simulink model "Controlador_NaoLinear_LQG"  (R2020a)
settings: Solver=ode8  StartTime=0.0  StopTime=50  FixedStep=0.01  RelTol=1e-3
values from neighbouring files (symbols this model uses):
  Ad = sysd.a    [Controlador.m]
  Bd = sysd.b    [Controlador.m]
  C = [1 0]    [Controlador.m]
  D = [0]    [Controlador.m]
  sysKFd = ss(Ad-Lf*C,[Bd Lf],eye(2),zeros(2,2))    [Controlador.m]
undefined symbols (not defined in the file or in its folder): kalmf, Krd
libraries: simulink x3
settings Model: Creator=Matheus  LastModifiedBy=mathe
settings DataIOCC: ReturnWorkspaceOutputs=off
settings DebuggingCC: ArithmeticOperatorsInVariantConditions=warning
settings SFSimCC: SimUseLocalCustomCode=off  CustomCodeUndefinedFunction=UseInterfaceOnly
settings RTWCC: RTWUseLocalCustomCode=off
settings CodeAppCC: StateflowObjectComments=on

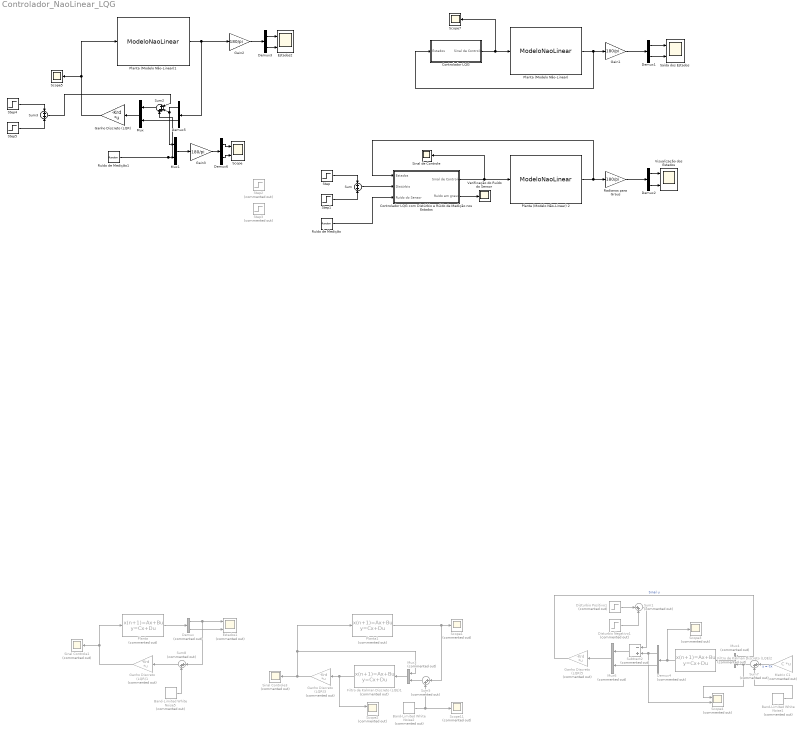
== system Controlador_NaoLinear_LQG ==
  Band-Limited White Noise1 : simulink/Sources/Band-Limited White Noise  Commented=on  Cov=0  Ts=0.05  seed=[23341]
  Band-Limited White Noise2 : simulink/Sources/Band-Limited White Noise  Commented=on  Cov=.0001  Ts=0.05  seed=[23341]
  Band-Limited White Noise5 : simulink/Sources/Band-Limited White Noise  Commented=on  Cov=.001  Ts=0.05  seed=[23341]
  Controlador LQG : Subsystem
  Controlador LQG com Distúrbio e Rúido de Medição nos Estados : Subsystem
  Demux : Demux  Commented=on  Outputs=2
  Demux{1..3,5..6} (5 alike) : Demux  Outputs=2
  Demux4 : Demux  Commented=on  Outputs=2
  Disturbio Negativo1 : Step  Commented=on  Time=10.5  After=-3.14/20
  Disturbio Positivo1 : Step  Commented=on  Time=10  After=3.14/20
  Estados1 : Scope  Commented=on  NumInputPorts=2
  Estados2 : Scope  NumInputPorts=2
  Filtro de Kalman Discreto (LQE)1 : DiscreteStateSpace  Commented=on  A=sysKFd.a  B=sysKFd.b  C=sysKFd.c  D=sysKFd.d  InitialCondition=[0 0]  SampleTime=0.05
  Filtro de Kalman Discreto (LQE)2 : DiscreteStateSpace  Commented=on  A=sysKFd.a  B=sysKFd.b  C=sysKFd.c  D=sysKFd.d  InitialCondition=[0 0]  SampleTime=-1
  Gain1 : Gain  Gain=180/pi
  Gain2 : Gain  Gain=180/pi
  Gain3 : Gain  Gain=180/pi
  Ganho Discreto (LQR) : Gain  Gain=-Krd  Multiplication=Matrix(K*u) (u vector)
  Ganho Discreto (LQR)1 : Gain  Commented=on  Gain=-Krd  Multiplication=Matrix(K*u) (u vector)
  Ganho Discreto (LQR)3 : Gain  Commented=on  Gain=-Krd  Multiplication=Matrix(K*u) (u vector)
  Ganho Discreto (LQR)5 : Gain  Commented=on  Gain=-Krd  Multiplication=Matrix(K*u) (u vector)
  Matriz C1 : Gain  Commented=on  Gain=C  Multiplication=Matrix(K*u) (u vector)
  Mux : Mux  Inputs=2
  Mux1 : Mux  Inputs=2
  Mux3 : Mux  Commented=on  Inputs=2
  Mux4 : Mux  Commented=on  Inputs=2
  Mux6 : Mux  Commented=on  Inputs=2
  Planta : DiscreteStateSpace  Commented=on  A=Ad  B=Bd  C=[eye(2); C]  D=[D; 0; 0]  InitialCondition=[pi/3 0]  SampleTime=0.05
  Planta (Modelo Não-Linear) : S-Function  InitFcn=try, set_param(gcb,'FunctionName','ModeloNaoLinear'), end  FunctionName=ModeloNaoLinear  SFunctionModules=ModeloNaoLinear_wrapper  SFunctionDeploymentMode=off  EnableBusSupport=off  mask(S-Function Builder){}
      mask help: Simulink:masks:SFunctionBuilder_MD
      mask init:
      | val = [[.9  0.75 0.75 1 1 .9 .9 1]',[1 1 0.75 0.75 .9 .9 1 .9]'];try , sys = get_param(gcb,'SfunBuilderFcnName');if isempty(sys), sys = get_param(gcb,'FunctionName'); end,catch, sys = get_param(gcb,'FunctionName'); end
      settings: CopyFcn=set_param(gcbh,'LinkStatus','none')  PreSaveFcn=try, set_param(gcb,'FunctionName','ModeloNaoLinear'), end  OpenFcn=sfunctionwizard(gcbh)
      mask Display: plot(val(:,1),val(:,2)),disp(sys), port_label('input',1,'u0'), port_label('output',1,'y0')
  Planta (Modelo Não-Linear) 2 : S-Function  InitFcn=try, set_param(gcb,'FunctionName','ModeloNaoLinear'), end  FunctionName=ModeloNaoLinear  SFunctionModules=ModeloNaoLinear_wrapper  SFunctionDeploymentMode=off  EnableBusSupport=off  mask(S-Function Builder){}
      mask help: Simulink:masks:SFunctionBuilder_MD
      mask init: same as Controlador_NaoLinear_LQG/Planta (Modelo Não-Linear)
      settings: CopyFcn=set_param(gcbh,'LinkStatus','none')  PreSaveFcn=try, set_param(gcb,'FunctionName','ModeloNaoLinear'), end  OpenFcn=sfunctionwizard(gcbh)
      mask Display: plot(val(:,1),val(:,2)),disp(sys), port_label('input',1,'u0'), port_label('output',1,'y0')
  Planta (Modelo Não-Linear)1 : S-Function  InitFcn=try, set_param(gcb,'FunctionName','ModeloNaoLinear'), end  FunctionName=ModeloNaoLinear  SFunctionModules=ModeloNaoLinear_wrapper  SFunctionDeploymentMode=off  EnableBusSupport=off  mask(S-Function Builder){}
      mask help: Simulink:masks:SFunctionBuilder_MD
      mask init: same as Controlador_NaoLinear_LQG/Planta (Modelo Não-Linear)
      settings: CopyFcn=set_param(gcbh,'LinkStatus','none')  PreSaveFcn=try, set_param(gcb,'FunctionName','ModeloNaoLinear'), end  OpenFcn=sfunctionwizard(gcbh)
      mask Display: plot(val(:,1),val(:,2)),disp(sys), port_label('input',1,'u0'), port_label('output',1,'y0')
  Planta1 : DiscreteStateSpace  Commented=on  A=Ad  B=Bd  C=C  D=D  InitialCondition=[pi/6 0]  SampleTime=0.05
  Radianos para Graus : Gain  Gain=180/pi
  Ruído de Medição : RandomNumber  Variance=0.0009  Seed=23341
  Ruído de Medição1 : RandomNumber  Variance=0.0009  Seed=23341
  Saída dos Estados : Scope  NumInputPorts=2
  Scope : Scope  NumInputPorts=2
  Scope1 : Scope  Commented=on
  Scope11 : Scope  Commented=on
  Scope2 : Scope  Commented=on  NumInputPorts=2
  Scope3 : Scope  Commented=on
  Scope4 : Scope  Commented=on  NumInputPorts=2
  Scope5 : Scope
  Scope7 : Scope
  Sinal Controle1 : Scope  Commented=on
  Sinal Controle3 : Scope  Commented=on
  Sinal de Controle : Scope
  Step : Step  Time=20  After=-0.0523599  SampleTime=0
  Step1 : Step  Time=20.5  After=0.0523599  SampleTime=0
  Step2 : Step  Commented=on  Time=15  After=-0.0523599  SampleTime=0
  Step3 : Step  Commented=on  Time=15.5  After=0.0523599  SampleTime=0
  Step4 : Step  Time=20  After=-0.0523599  SampleTime=0
  Step5 : Step  Time=20.5  After=0.0523599  SampleTime=0
  Subtract2 : Sum  Commented=on  Inputs=-+
  Sum : Sum
  Sum{1,5,7..8} (4 alike) : Sum  Commented=on  Inputs=|++
  Sum2 : Sum  Inputs=|+++
  Sum3 : Sum
  Verificação do Ruído do Sensor : Scope
  Visualização dos Estados : Scope  NumInputPorts=2
  wires:
  Ganho Discreto (LQR)/1 -> Scope5/1, Planta (Modelo Não-Linear)1/1
  Planta (Modelo Não-Linear)1/1 -> Demux5/1, Gain2/1
  Planta/1 -> Demux/1
  Demux/1 -> Sum8/1, Estados1/1
  Ganho Discreto (LQR)1/1 -> Planta/1, Sinal Controle1/1
  Mux3/1 -> Filtro de Kalman Discreto (LQE)1/1
  Planta1/1 -> Sum5/1, Scope1/1
  Sum5/1 -> Mux3/2
  Demux/2 -> Estados1/2
  Band-Limited White Noise2/1 -> Scope11/1, Sum5/2
  Filtro de Kalman Discreto (LQE)1/1 -> Scope2/1, Ganho Discreto (LQR)3/1
  Ganho Discreto (LQR)3/1 -> Planta1/1, Mux3/1, Sinal Controle3/1
  Sum8/1 -> Ganho Discreto (LQR)1/1
  Band-Limited White Noise5/1 -> Sum8/2
  Demux4/2 -> Mux6/2
  Sum1/1 -> Subtract2/1
  Subtract2/1 -> Mux6/1
  Ganho Discreto (LQR)5/1 -> Mux4/1  "Sinal u"
  Disturbio Negativo1/1 -> Sum1/2
  Mux4/1 -> Filtro de Kalman Discreto (LQE)2/1
  Matriz C1/1 -> Sum7/1  "y = Cx"
  Band-Limited White Noise1/1 -> Sum7/2
  Sum7/1 -> Scope4/1, Mux4/2
  Filtro de Kalman Discreto (LQE)2/1 -> Scope3/1, Demux4/1
  Mux6/1 -> Ganho Discreto (LQR)5/1
  Demux4/1 -> Scope4/2, Subtract2/2
  Disturbio Positivo1/1 -> Sum1/1
  Gain1/1 -> Demux1/1
  Demux1/2 -> Saída dos Estados/2
  Demux1/1 -> Saída dos Estados/1
  Controlador LQG com Distúrbio e Rúido de Medição nos Estados/1(Sinal de Controle) -> Sinal de Controle/1, Planta (Modelo Não-Linear) 2/1
  Ruído de Medição/1 -> Controlador LQG com Distúrbio e Rúido de Medição nos Estados/3(Ruído do Sensor)
  Controlador LQG com Distúrbio e Rúido de Medição nos Estados/2(Ruído em graus) -> Verificação do Ruído do Sensor/1
  Radianos para Graus/1 -> Demux2/1
  Demux2/1 -> Visualização dos Estados/1
  Demux2/2 -> Visualização dos Estados/2
  Step1/1 -> Sum/2
  Step/1 -> Sum/1
  Sum/1 -> Controlador LQG com Distúrbio e Rúido de Medição nos Estados/2(Distúrbio)
  Gain2/1 -> Demux3/1
  Demux3/1 -> Estados2/1
  Mux/1 -> Ganho Discreto (LQR)/1
  Demux5/2 -> Mux/2
  Sum2/1 -> Mux/1
  Demux5/1 -> Sum2/2, Mux1/1
  Ruído de Medição1/1 -> Sum2/3, Mux1/2
  Gain3/1 -> Demux6/1
  Demux6/2 -> Scope/2
  Demux6/1 -> Scope/1
  Mux1/1 -> Gain3/1
  Planta (Modelo Não-Linear)/1 -> Controlador LQG/1(Estados), Gain1/1
  Controlador LQG/1(Sinal de Controle) -> Scope7/1, Planta (Modelo Não-Linear)/1
  Planta (Modelo Não-Linear) 2/1 -> Controlador LQG com Distúrbio e Rúido de Medição nos Estados/1(Estados), Radianos para Graus/1
  Demux3/2 -> Estados2/2
  Step4/1 -> Sum3/1
  Step5/1 -> Sum3/2
  Sum3/1 -> Sum2/1

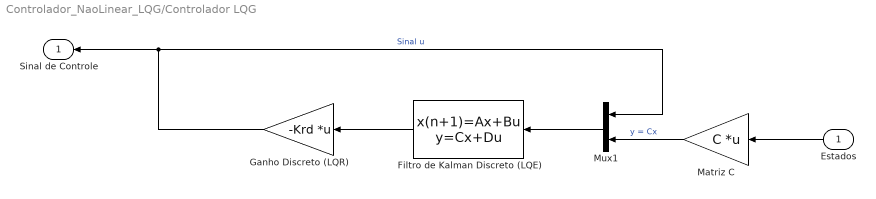
== system Controlador_NaoLinear_LQG/Controlador LQG ==
  Estados : Inport
  Filtro de Kalman Discreto (LQE) : DiscreteStateSpace  A=sysKFd.a  B=sysKFd.b  C=sysKFd.c  D=sysKFd.d  InitialCondition=[0 0]  SampleTime=-1
  Ganho Discreto (LQR) : Gain  Gain=-Krd  Multiplication=Matrix(K*u) (u vector)
  Matriz C : Gain  Gain=C  Multiplication=Matrix(K*u) (u vector)
  Mux1 : Mux  Inputs=2
  Sinal de Controle : Outport
  wires:
  Filtro de Kalman Discreto (LQE)/1 -> Ganho Discreto (LQR)/1
  Matriz C/1 -> Mux1/2  "y = Cx"
  Ganho Discreto (LQR)/1 -> Sinal de Controle/1, Mux1/1  "Sinal u"
  Estados/1 -> Matriz C/1
  Mux1/1 -> Filtro de Kalman Discreto (LQE)/1

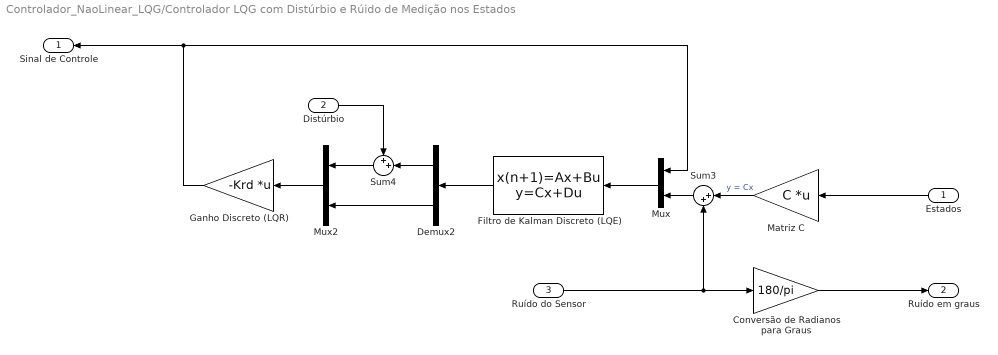
== system Controlador_NaoLinear_LQG/Controlador LQG com Distúrbio e Rúido de Medição nos Estados ==
  Estados : Inport
  Distúrbio : Inport  Port=2
  Ruído do Sensor : Inport  Port=3
  Conversão de Radianos para Graus : Gain  Gain=180/pi
  Demux2 : Demux  Outputs=2
  Filtro de Kalman Discreto (LQE) : DiscreteStateSpace  A=kalmf.a  B=[Bd kalmf.b]  C=eye(2)  D=zeros(2,2)  InitialCondition=[0 0]  SampleTime=-1
  Ganho Discreto (LQR) : Gain  Gain=-Krd  Multiplication=Matrix(K*u) (u vector)
  Matriz C : Gain  Gain=C  Multiplication=Matrix(K*u) (u vector)
  Mux : Mux  Inputs=2
  Mux2 : Mux  Inputs=2
  Sum3 : Sum  Inputs=|++
  Sum4 : Sum  Inputs=++|
  Sinal de Controle : Outport
  Ruído em graus : Outport  Port=2
  wires:
  Ruído do Sensor/1 -> Conversão de Radianos para Graus/1, Sum3/2
  Mux2/1 -> Ganho Discreto (LQR)/1
  Mux/1 -> Filtro de Kalman Discreto (LQE)/1
  Sum3/1 -> Mux/2
  Matriz C/1 -> Sum3/1  "y = Cx"
  Filtro de Kalman Discreto (LQE)/1 -> Demux2/1
  Demux2/2 -> Mux2/2
  Ganho Discreto (LQR)/1 -> Sinal de Controle/1, Mux/1
  Conversão de Radianos para Graus/1 -> Ruído em graus/1
  Distúrbio/1 -> Sum4/1
  Demux2/1 -> Sum4/2
  Sum4/1 -> Mux2/1
  Estados/1 -> Matriz C/1
